simulink subsystem "Voltage_Eq"  (R2022b)
settings: Solver=VariableStepAuto  StartTime=0.0  StopTime=10.0  RelTol=1e-3
model mask{R=R, Ls=Ls, Lr=Lr}
  mask prompts: R "Stator Resistance (R)"; Ls "Stator Inductance (Ls)"; Lr "Rotor Inductance (Lr)"
settings Model: Creator=MAAM  LastModifiedBy=MAAM

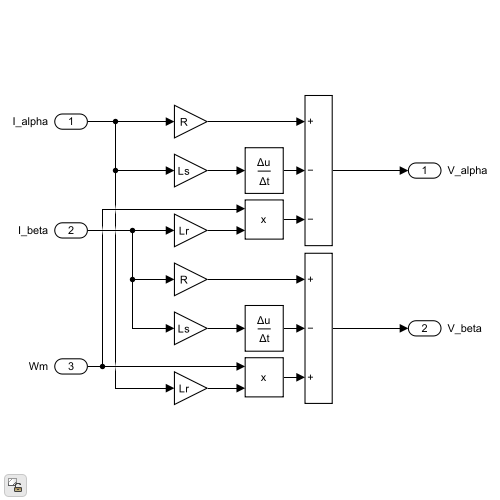
[thumbnail: Simulink's stored preview of the top-level diagram]
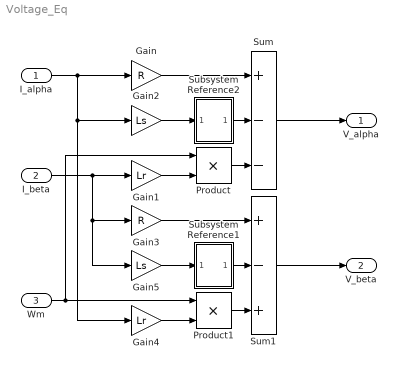
== system Voltage_Eq ==
  I_alpha : Inport
  I_beta : Inport  Port=2
  Wm : Inport  Port=3
  Gain : Gain  Gain=R
  Gain1 : Gain  Gain=Lr
  Gain2 : Gain  Gain=Ls
  Gain3 : Gain  Gain=R
  Gain4 : Gain  Gain=Lr
  Gain5 : Gain  Gain=Ls
  Product : Product
  Product1 : Product
  Subsystem Reference1 : Subsystem  ReferencedSubsystem=Derivative  Gain=1.0  Init=0  SampleTime=-1  Ts=0.001
  Subsystem Reference2 : Subsystem  ReferencedSubsystem=Derivative  Gain=1.0  Init=0  SampleTime=-1  Ts=0.001
  Sum : Sum  Inputs=+--
  Sum1 : Sum  Inputs=+-+
  V_alpha : Outport
  V_beta : Outport  Port=2
  wires:
  Sum/1 -> V_alpha/1
  Product/1 -> Sum/3
  I_alpha/1 -> Gain4/1, Gain2/1, Gain/1
  Gain/1 -> Sum/1
  Subsystem Reference2/1 -> Sum/2
  Gain2/1 -> Subsystem Reference2/1
  Gain1/1 -> Product/2
  Gain4/1 -> Product1/2
  Gain5/1 -> Subsystem Reference1/1
  Subsystem Reference1/1 -> Sum1/2
  Gain3/1 -> Sum1/1
  I_beta/1 -> Gain1/1, Gain3/1, Gain5/1
  Product1/1 -> Sum1/3
  Wm/1 -> Product1/1, Product/1
  Sum1/1 -> V_beta/1
